simulink model "Stryfe_Simulation"  (R2020b)
settings: Solver=VariableStepAuto  StartTime=0.0  StopTime=3.75  RelTol=1e-3
libraries: simulink_extras x3, simulink x2, shared3dof x1, pid_lib x1
settings Model: Creator=Jacob  LastModifiedBy=bowen

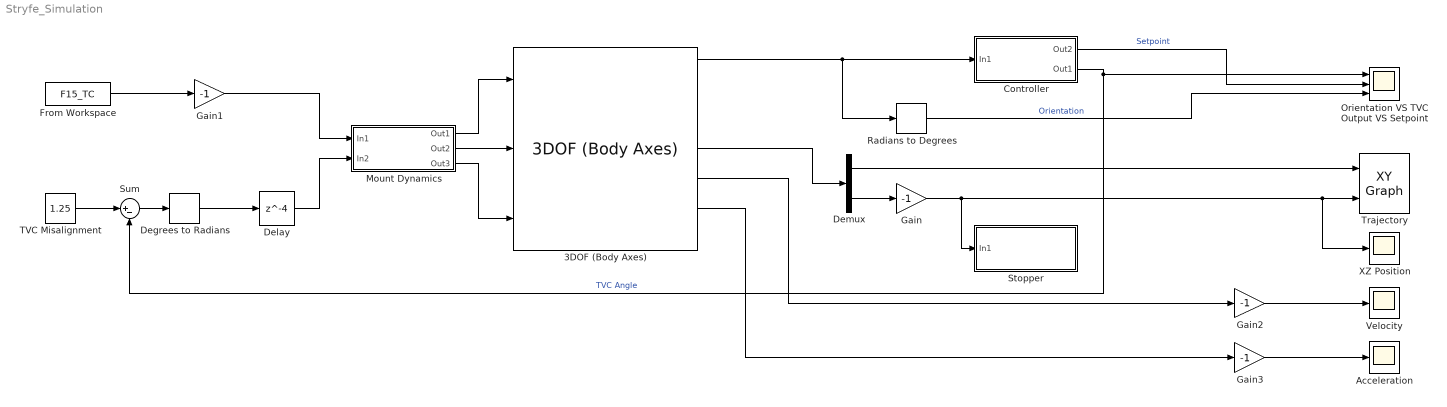
== system Stryfe_Simulation ==
  3DOF (Body Axes) : shared3dof/3DOF (Body Axes)  units=Metric (MKS)  mtype=Fixed  v_ini=0  theta_ini=0  alpha_ini=0  pos_ini=[0 0]  q_ini=0  mass=0.726  mass_e=0.450  mass_f=0.485  Iyy=0.06926426849  Iyy_e=0.1736  Iyy_f=0.18756  g_in=Internal  g=9.81  vre_flag=on  abi_flag=on  aMode=0  vel_statename=''  theta_statename=''  pos_statename=''  q_statename=''  mass_statename=''
      settings: SourceProductBaseCode=AE,PW,MT,UV,VE,VP
  Acceleration : Scope
  Controller : Subsystem
  Degrees to Radians : simulink_extras/Transformations/Degrees to Radians
  Delay : Delay  DelayLength=4  SampleTime=0.01
  Demux : Demux  Outputs=2
  From Workspace : FromWorkspace  VariableName=F15_TC
  Gain{,1..3} (4 alike) : Gain  Gain=-1
  Mount Dynamics : Subsystem
  Orientation VS TVC Output VS Setpoint : Scope  NumInputPorts=3
  Radians to Degrees : simulink_extras/Transformations/Radians to Degrees
  Stopper : Subsystem
  Sum : Sum  Inputs=|+-
  TVC Misalignment : Constant  Value=1.25
  Trajectory : simulink/Sinks/XY Graph  xmin=-20  xmax=20  ymin=-1  ymax=125  st=-1
  Velocity : Scope
  XZ Position : Scope
  wires:
  Demux/2 -> Gain/1
  Gain/1 -> Stopper/1(In1), XZ Position/1, Trajectory/2
  TVC Misalignment/1 -> Sum/1
  Controller/2(Out1) -> Orientation VS TVC Output VS Setpoint/1, Sum/2  "TVC Angle"
  3DOF (Body Axes)/6 -> Gain3/1
  3DOF (Body Axes)/5 -> Gain2/1
  Demux/1 -> Trajectory/1
  3DOF (Body Axes)/4 -> Demux/1
  From Workspace/1 -> Gain1/1
  Mount Dynamics/1(Out1) -> 3DOF (Body Axes)/1
  Mount Dynamics/2(Out2) -> 3DOF (Body Axes)/2
  Mount Dynamics/3(Out3) -> 3DOF (Body Axes)/3
  Sum/1 -> Degrees to Radians/1
  Controller/1(Out2) -> Orientation VS TVC Output VS Setpoint/2  "Setpoint"
  Radians to Degrees/1 -> Orientation VS TVC Output VS Setpoint/3  "Orientation"
  Degrees to Radians/1 -> Delay/1
  Delay/1 -> Mount Dynamics/2(In2)
  Gain1/1 -> Mount Dynamics/1(In1)
  Gain2/1 -> Velocity/1
  Gain3/1 -> Acceleration/1
  3DOF (Body Axes)/1 -> Radians to Degrees/1, Controller/1(In1)

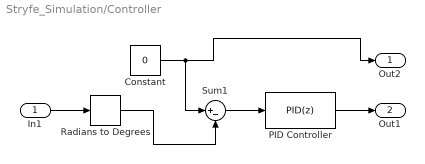
== system Stryfe_Simulation/Controller ==
  In1 : Inport
  Constant : Constant  Value=0
  PID Controller : pid_lib/PID Controller  Controller=PID  Form=Parallel  TimeDomain=Discrete-time  UseExternalTs=off  SampleTime=0.025  IntegratorMethod=Forward Euler  FilterMethod=Forward Euler  ControllerParametersSource=internal  P=0.6  I=0.155  D=0.14  UseFilter=off  N=100  TunerSelectOption=Transfer Function Based (PID Tuner App)  InitialConditionSource=internal  InitialConditionForIntegrator=0  InitialConditionForFilter=0  DifferentiatorICPrevScaledInput=0  ExternalReset=none  TrackingMode=off  Kt=1  LimitOutput=on  SatLimitsSource=internal  UpperSaturationLimit=5  LowerSaturationLimit=-5  LinearizeAsGain=off  AntiWindupMode=clamping  Kb=1  POutMin=[]  POutMax=[]  IOutMin=[]  IOutMax=[]  DOutMin=[]  DOutMax=[]  NOutMin=[]  NOutMax=[]  SumOutMin=[]  SumOutMax=[]  SaturationOutMin=[]  SaturationOutMax=[]  PParamMin=[]  PParamMax=[]  IParamMin=[]  IParamMax=[]  DParamMin=[]  DParamMax=[]  NParamMin=[]  NParamMax=[]  KbParamMin=[]  KbParamMax=[]  KtParamMin=[]  KtParamMax=[]  KbOutMin=[]  KbOutMax=[]  KtOutMin=[]  KtOutMax=[]  IntegratorOutMin=[]  IntegratorOutMax=[]  FilterOutMin=[]  FilterOutMax=[]  SumI1OutMin=[]  SumI1OutMax=[]  SumI2OutMin=[]  SumI2OutMax=[]  SumI3OutMin=[]  SumI3OutMax=[]  SumI4OutMin=[]  SumI4OutMax=[]  SumDOutMin=[]  SumDOutMax=[]  DifferentiatorOutMin=[]  DifferentiatorOutMax=[]  FilterDiffOutCoefMin=[]  FilterDiffOutCoefMax=[]  ReciprocalOutMin=[]  ReciprocalOutMax=[]  SumDenOutMin=[]  SumDenOutMax=[]  SumNumOutMin=[]  SumNumOutMax=[]  DivideOutMin=[]  DivideOutMax=[]  UdiffTsProdOutMin=[]  UdiffTsProdOutMax=[]  NTsProdOutMin=[]  NTsProdOutMax=[]  UintegralTsProdOutMin=[]  UintegralTsProdOutMax=[]  UngainTsProdOutMin=[]  UngainTsProdOutMax=[]  IntegratorContinuousStateAttributes=''  IntegratorStateMustResolveToSignalObject=off  IntegratorRTWStateStorageClass=Auto  FilterContinuousStateAttributes=''  FilterStateMustResolveToSignalObject=off  FilterRTWStateStorageClass=Auto  ParallelPVariant=InternalParameters  IdealPVariant=Disabled  IVariant=InternalParameters  DVariant=InternalParameters  IntegratorVariant=Discrete  SatVariant=Enabled  AWVariant=DiscClampingParallel  PCopyVariant=Disabled  TRVariant=Disabled  FdbkBlocksVariant=Forward  IdealPFdbkVariant=Disabled  SatFdbkVariant=Disabled  DerivativeFilterVariant=Differentiator  NVariant=Passthrough  NCopyVariant=Disabled_SignalSpec  FilterICVariant=InternalICsDifferentiator  IntegratorICVariant=InternalICs  ExternalResetVariant=Disabled  TRSumVariant=Passthrough  SumFdbkVariant=Disabled  SumVariant=Sum_PID  TsampFilterVariant=InternalTs  TsampNgainVariant=Passthrough  TsampIntegralVariant=Passthrough  ExternalSaturationOutDataTypeStr=Inherit: Same as second input
  Radians to Degrees : simulink_extras/Transformations/Radians to Degrees
  Sum1 : Sum  Inputs=|+-
  Out2 : Outport
  Out1 : Outport  Port=2
  wires:
  In1/1 -> Radians to Degrees/1
  Constant/1 -> Out2/1, Sum1/1
  Radians to Degrees/1 -> Sum1/2
  PID Controller/1 -> Out1/1
  Sum1/1 -> PID Controller/1

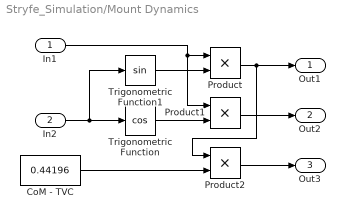
== system Stryfe_Simulation/Mount Dynamics ==
  In1 : Inport
  In2 : Inport  Port=2
  CoM - TVC : Constant  Value=0.44196
  Product : Product
  Product1 : Product
  Product2 : Product
  Trigonometric Function : Trigonometry  Operator=cos
  Trigonometric Function1 : Trigonometry
  Out1 : Outport
  Out2 : Outport  Port=2
  Out3 : Outport  Port=3
  wires:
  In1/1 -> Product1/1, Product/1
  Trigonometric Function1/1 -> Product/2
  Product/1 -> Out1/1, Product2/1
  CoM - TVC/1 -> Product2/2
  Trigonometric Function/1 -> Product1/2
  In2/1 -> Trigonometric Function/1, Trigonometric Function1/1
  Product2/1 -> Out3/1
  Product1/1 -> Out2/1

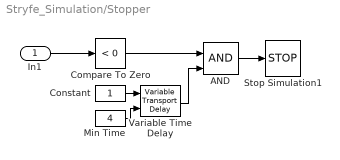
== system Stryfe_Simulation/Stopper ==
  In1 : Inport
  AND : Logic  IconShape=distinctive  AllPortsSameDT=off  OutDataTypeStr=boolean
  Compare To Zero : simulink/Logic and Bit Operations/Compare To Zero  relop=<  OutDataTypeStr=boolean
  Constant : Constant
  Min Time : Constant  Value=4
  Stop Simulation1 : Stop
  Variable Time Delay : VariableTransportDelay  MaximumDelay=10
  wires:
  Compare To Zero/1 -> AND/1
  AND/1 -> Stop Simulation1/1
  Constant/1 -> Variable Time Delay/1
  Variable Time Delay/1 -> AND/2
  Min Time/1 -> Variable Time Delay/2
  In1/1 -> Compare To Zero/1
